simulink model "W2ques3_system"  (R2020b)
settings: Solver=VariableStepAuto  StartTime=0.0  StopTime=10.0  RelTol=1e-3
values from neighbouring files (symbols this model uses):
  b = 50.0    [DataDict_Cruise.sldd]    (also in W2ques3_code.m = 50)
  m = 1000.0    [DataDict_Cruise.sldd]    (also in W2ques3_code.m = 1000)
settings Model: Creator=sneha  LastModifiedBy=sneha

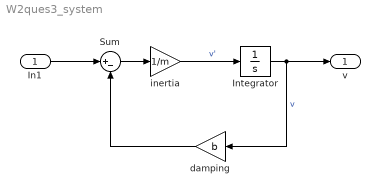
== system W2ques3_system ==
  In1 : Inport
  Integrator : Integrator
  Sum : Sum  Inputs=|+-
  damping : Gain  Gain=b
  inertia : Gain  Gain=1/m
  v : Outport
  wires:
  In1/1 -> Sum/1
  Sum/1 -> inertia/1
  Integrator/1 -> v/1, damping/1  "v"
  inertia/1 -> Integrator/1  "v'"
  damping/1 -> Sum/2
